simulink model "AutoRS_Simulink"  (R2022b)
settings: Solver=FixedStepAuto  StartTime=0.0  StopTime=50  FixedStep=1e-4  RelTol=1e-3
values from neighbouring files (symbols this model uses):
  c = Konstanten()    [AutoRS.m]
settings Model: Creator=Sebastian  LastModifiedBy=Sebastian

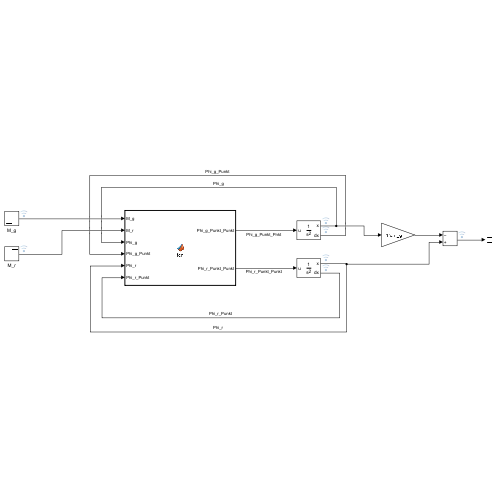
[thumbnail: Simulink's stored preview of the top-level diagram]
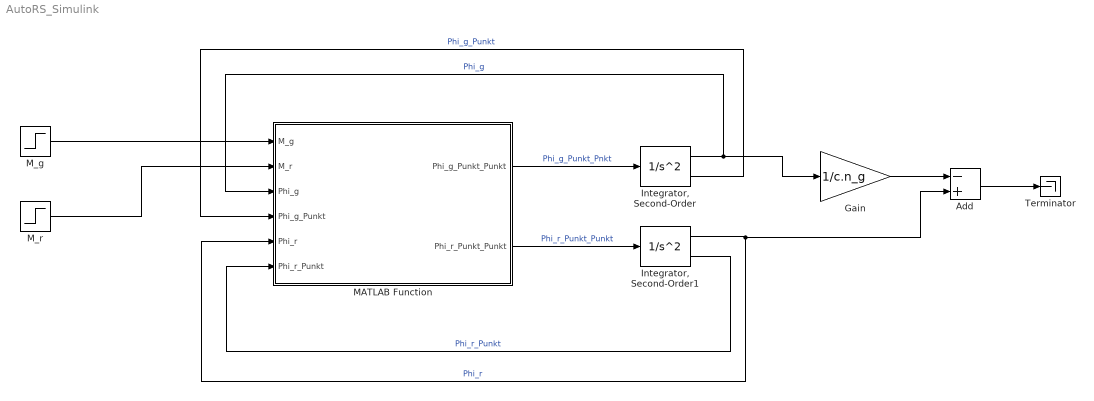
== system AutoRS_Simulink ==
  Add : Sum  Inputs=-+
  Gain : Gain  Gain=1/c.n_g
  "Integrator, Second-Order" : SecondOrderIntegrator
  "Integrator, Second-Order1" : SecondOrderIntegrator
  MATLAB Function : MATLAB Function  TreatAsAtomicUnit=on
  M_g : Step  Time=15  After=(1/c.n_g)*100  SampleTime=0
  M_r : Step  Time=5  After=100  SampleTime=0
  Terminator : Terminator
  wires:
  MATLAB Function/2(Phi_r_Punkt_Punkt) -> "Integrator, Second-Order1"/1  "Phi_r_Punkt_Punkt"
  MATLAB Function/1(Phi_g_Punkt_Punkt) -> "Integrator, Second-Order"/1  "Phi_g_Punkt_Pnkt"
  "Integrator, Second-Order"/2 -> MATLAB Function/4(Phi_g_Punkt)  "Phi_g_Punkt"
  "Integrator, Second-Order"/1 -> Gain/1, MATLAB Function/3(Phi_g)  "Phi_g"
  "Integrator, Second-Order1"/2 -> MATLAB Function/6(Phi_r_Punkt)  "Phi_r_Punkt"
  "Integrator, Second-Order1"/1 -> Add/2, MATLAB Function/5(Phi_r)  "Phi_r"
  M_g/1 -> MATLAB Function/1(M_g)
  M_r/1 -> MATLAB Function/2(M_r)
  Gain/1 -> Add/1
  Add/1 -> Terminator/1

== matlab function AutoRS_Simulink/MATLAB Function ==
  data: M_g input; M_r input; Phi_g_Punkt_Punkt output; Phi_r_Punkt_Punkt output; Phi_g input; Phi_g_Punkt input; Phi_r input; Phi_r_Punkt input
function [Phi_g_Punkt_Punkt, Phi_r_Punkt_Punkt]= fcn(M_g, M_r, Phi_g, Phi_g_Punkt, Phi_r, Phi_r_Punkt)

    c = Konstanten();

    Phi_g_Punkt_Punkt = (-c.k_s*(Phi_g-c.n_g*Phi_r)-c.d_s*(Phi_g_Punkt-c.n_g*Phi_r_Punkt)-M_g)/c.J_g;

    Phi_r_Punkt_Punkt = (M_r-c.n_g*(c.k_s*(c.n_g*Phi_r-Phi_g))-c.n_g*(c.d_s*(c.n_g*Phi_r_Punkt-Phi_g_Punkt)))/c.J_r;

end
